simulink model "Quad_Linear_Openloop_LQDG"  (R2020a)
settings: Solver=ode4  StartTime=0.0  StopTime=15  FixedStep=0.01  RelTol=1e-3
InitFcn:
  | OpenLoop_LQDG_riccati_solver
undefined symbols (not defined in the file): A1, A3, B1, B3, C2, LQDG_openloop_gain, Omega, x0
settings Model: Creator=Ali  LastModifiedBy=Ali

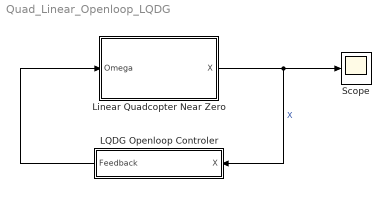
== system Quad_Linear_Openloop_LQDG ==
  LQDG Openloop Controler : Subsystem
  Linear Quadcopter Near Zero : Subsystem
  Scope : Scope
  wires:
  Linear Quadcopter Near Zero/1(X) -> Scope/1, LQDG Openloop Controler/1(X)  "X"
  LQDG Openloop Controler/1(Feedback) -> Linear Quadcopter Near Zero/1(Omega)

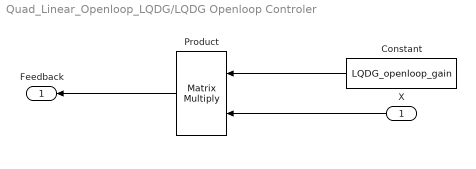
== system Quad_Linear_Openloop_LQDG/LQDG Openloop Controler ==
  X : Inport
  Constant : Constant  Value=LQDG_openloop_gain
  Product : Product  Multiplication=Matrix(*)
  Feedback : Outport
  wires:
  Product/1 -> Feedback/1
  X/1 -> Product/2
  Constant/1 -> Product/1

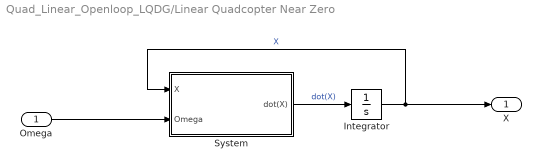
== system Quad_Linear_Openloop_LQDG/Linear Quadcopter Near Zero ==
  Omega : Inport
  Integrator : Integrator  InitialCondition=x0
  System : Subsystem
  X : Outport
  wires:
  Integrator/1 -> X/1, System/1(X)  "X"
  System/1(dot(X)) -> Integrator/1  "dot(X)"
  Omega/1 -> System/2(Omega)

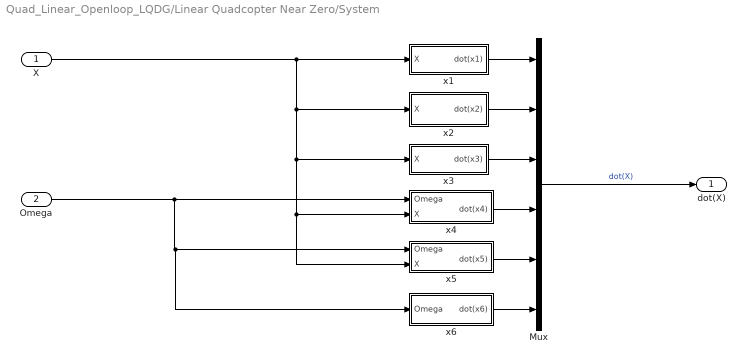
== system Quad_Linear_Openloop_LQDG/Linear Quadcopter Near Zero/System ==
  X : Inport
  Omega : Inport  Port=2
  Mux : Mux  Inputs=6
  x1 : Subsystem
  x2 : Subsystem
  x3 : Subsystem
  x4 : Subsystem
  x5 : Subsystem
  x6 : Subsystem
  dot(X) : Outport
  wires:
  Omega/1 -> x4/1(Omega), x6/1(Omega), x5/1(Omega)
  x6/1(dot(x6)) -> Mux/6
  x3/1(dot(x3)) -> Mux/3
  x4/1(dot(x4)) -> Mux/4
  x2/1(dot(x2)) -> Mux/2
  X/1 -> x5/2(X), x4/2(X), x3/1(X), x2/1(X), x1/1(X)
  x5/1(dot(x5)) -> Mux/5
  x1/1(dot(x1)) -> Mux/1
  Mux/1 -> dot(X)/1  "dot(X)"

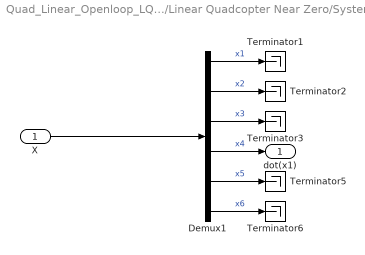
== system Quad_Linear_Openloop_LQDG/Linear Quadcopter Near Zero/System/x1 ==
  X : Inport
  Demux1 : Demux  Outputs=6
  Terminator{1..3,5..6} (5 alike) : Terminator
  dot(x1) : Outport
  wires:
  Demux1/4 -> dot(x1)/1  "x4"
  X/1 -> Demux1/1
  Demux1/6 -> Terminator6/1  "x6"
  Demux1/5 -> Terminator5/1  "x5"
  Demux1/3 -> Terminator3/1  "x3"
  Demux1/2 -> Terminator2/1  "x2"
  Demux1/1 -> Terminator1/1  "x1"

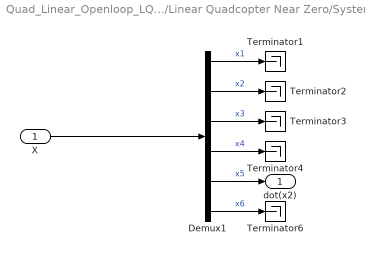
== system Quad_Linear_Openloop_LQDG/Linear Quadcopter Near Zero/System/x2 ==
  X : Inport
  Demux1 : Demux  Outputs=6
  Terminator{1..4,6} (5 alike) : Terminator
  dot(x2) : Outport
  wires:
  Demux1/4 -> Terminator4/1  "x4"
  X/1 -> Demux1/1
  Demux1/6 -> Terminator6/1  "x6"
  Demux1/5 -> dot(x2)/1  "x5"
  Demux1/3 -> Terminator3/1  "x3"
  Demux1/2 -> Terminator2/1  "x2"
  Demux1/1 -> Terminator1/1  "x1"

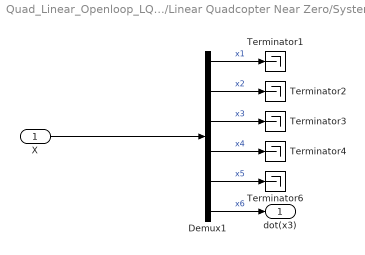
== system Quad_Linear_Openloop_LQDG/Linear Quadcopter Near Zero/System/x3 ==
  X : Inport
  Demux1 : Demux  Outputs=6
  Terminator{1..4,6} (5 alike) : Terminator
  dot(x3) : Outport
  wires:
  Demux1/4 -> Terminator4/1  "x4"
  X/1 -> Demux1/1
  Demux1/6 -> dot(x3)/1  "x6"
  Demux1/5 -> Terminator6/1  "x5"
  Demux1/3 -> Terminator3/1  "x3"
  Demux1/2 -> Terminator2/1  "x2"
  Demux1/1 -> Terminator1/1  "x1"

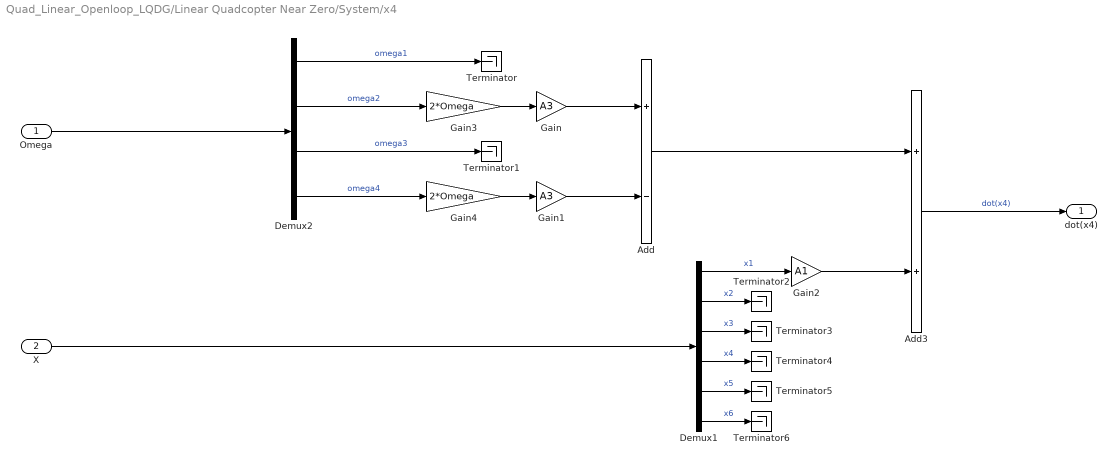
== system Quad_Linear_Openloop_LQDG/Linear Quadcopter Near Zero/System/x4 ==
  Omega : Inport
  X : Inport  Port=2
  Add : Sum  Inputs=+-
  Add3 : Sum
  Demux1 : Demux  Outputs=6
  Demux2 : Demux
  Gain : Gain  Gain=A3
  Gain1 : Gain  Gain=A3
  Gain2 : Gain  Gain=A1
  Gain3 : Gain  Gain=2*Omega
  Gain4 : Gain  Gain=2*Omega
  Terminator{,1..6} (7 alike) : Terminator
  dot(x4) : Outport
  wires:
  Gain2/1 -> Add3/2
  Gain1/1 -> Add/2
  Gain/1 -> Add/1
  Demux2/4 -> Gain4/1  "omega4"
  Demux2/2 -> Gain3/1  "omega2"
  Demux2/3 -> Terminator1/1  "omega3"
  Demux2/1 -> Terminator/1  "omega1"
  Demux1/5 -> Terminator5/1  "x5"
  Demux1/2 -> Terminator2/1  "x2"
  Demux1/3 -> Terminator3/1  "x3"
  Demux1/1 -> Gain2/1  "x1"
  Demux1/4 -> Terminator4/1  "x4"
  X/1 -> Demux1/1
  Demux1/6 -> Terminator6/1  "x6"
  Gain3/1 -> Gain/1
  Gain4/1 -> Gain1/1
  Omega/1 -> Demux2/1
  Add/1 -> Add3/1
  Add3/1 -> dot(x4)/1  "dot(x4)"

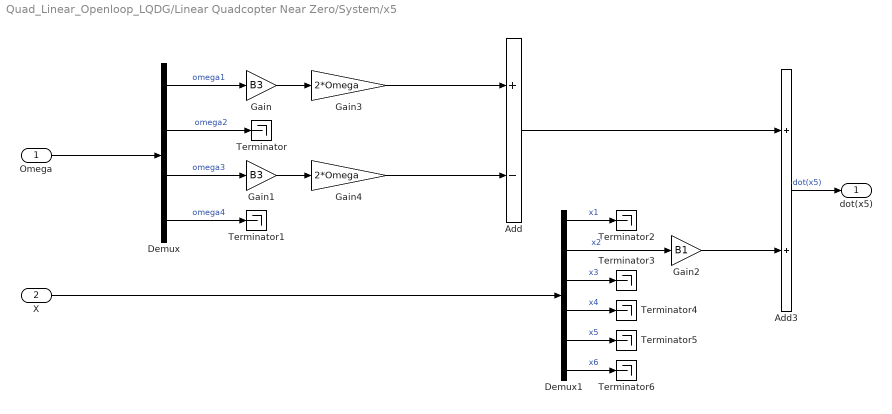
== system Quad_Linear_Openloop_LQDG/Linear Quadcopter Near Zero/System/x5 ==
  Omega : Inport
  X : Inport  Port=2
  Add : Sum  Inputs=+-
  Add3 : Sum
  Demux : Demux
  Demux1 : Demux  Outputs=6
  Gain : Gain  Gain=B3
  Gain1 : Gain  Gain=B3
  Gain2 : Gain  Gain=B1
  Gain3 : Gain  Gain=2*Omega
  Gain4 : Gain  Gain=2*Omega
  Terminator{,1..6} (7 alike) : Terminator
  dot(x5) : Outport
  wires:
  Gain1/1 -> Gain4/1
  Gain/1 -> Gain3/1
  Demux/2 -> Terminator/1  "omega2"
  Demux/4 -> Terminator1/1  "omega4"
  Demux/1 -> Gain/1  "omega1"
  Demux/3 -> Gain1/1  "omega3"
  Demux1/5 -> Terminator5/1  "x5"
  Demux1/2 -> Gain2/1  "x2"
  Demux1/3 -> Terminator3/1  "x3"
  Demux1/1 -> Terminator2/1  "x1"
  Demux1/4 -> Terminator4/1  "x4"
  X/1 -> Demux1/1
  Demux1/6 -> Terminator6/1  "x6"
  Gain3/1 -> Add/1
  Gain4/1 -> Add/2
  Omega/1 -> Demux/1
  Add/1 -> Add3/1
  Gain2/1 -> Add3/2
  Add3/1 -> dot(x5)/1  "dot(x5)"

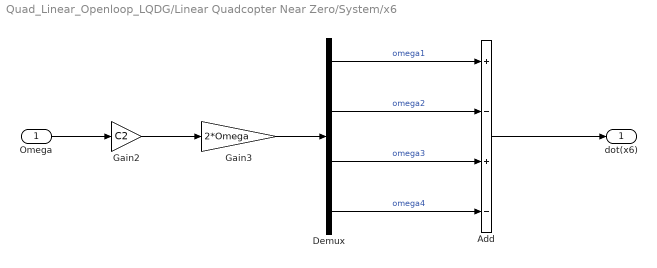
== system Quad_Linear_Openloop_LQDG/Linear Quadcopter Near Zero/System/x6 ==
  Omega : Inport
  Add : Sum  Inputs=+-+-
  Demux : Demux
  Gain2 : Gain  Gain=C2
  Gain3 : Gain  Gain=2*Omega
  dot(x6) : Outport
  wires:
  Omega/1 -> Gain2/1
  Demux/1 -> Add/1  "omega1"
  Demux/2 -> Add/2  "omega2"
  Demux/3 -> Add/3  "omega3"
  Demux/4 -> Add/4  "omega4"
  Add/1 -> dot(x6)/1
  Gain3/1 -> Demux/1
  Gain2/1 -> Gain3/1
